simulink model "signalSim"  (R2023b)
settings: Solver=VariableStepAuto  StartTime=0.0  StopTime=0.1  RelTol=1e-3
values from neighbouring files (symbols this model uses):
  f = 1000    [data_gen.m]    (also in test.m = 100)
  fdac = 20e6    (= 20000000)    [data_gen.m]
  fs = 1e6    (= 1000000)    [data_gen.m]    (also in test.m = 1000)
  inc_1e5 = round((100000*2^N)/fdac)    [data_gen.m]
libraries: hdlsllib x3, dspsrcs4 x2, dspfdesign x1, dsphdlsigops2 x1
settings Model: Creator=31651  LastModifiedBy=31651
settings OptimizationCC: BlockReduction=off  ConditionallyExecuteInputs=off

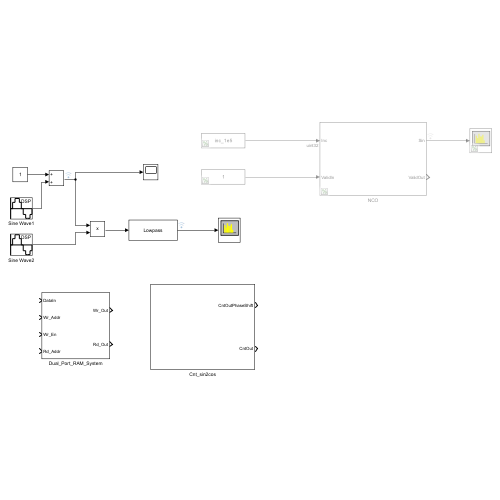
[thumbnail: Simulink's stored preview of the top-level diagram]
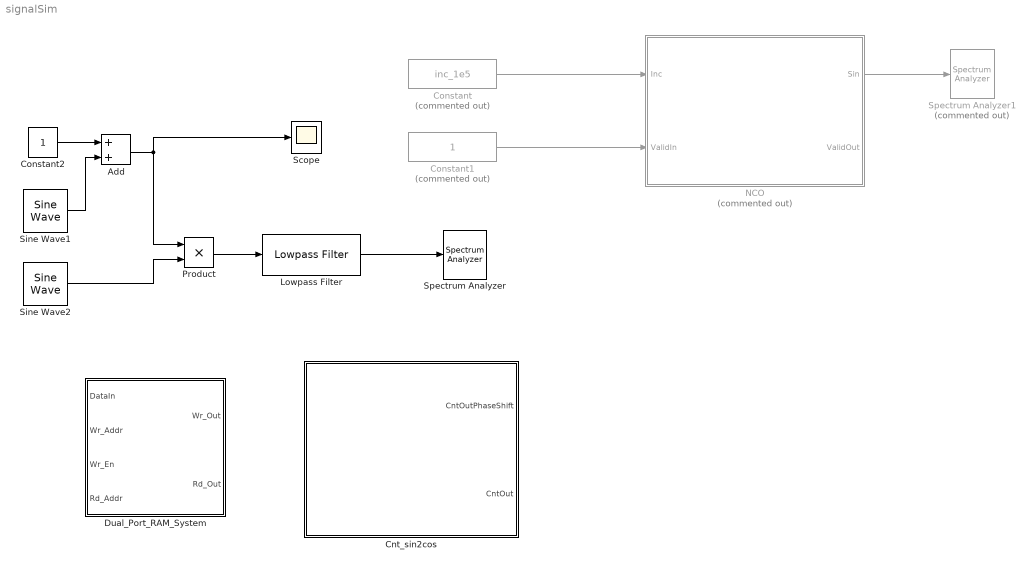
== system signalSim ==
  Add : Sum
  Cnt_sin2cos : Subsystem
  Constant : Constant  Commented=on  Value=inc_1e5  OutDataTypeStr=uint32  SampleTime=1/fdac
  Constant1 : Constant  Commented=on  OutDataTypeStr=boolean  SampleTime=1/fdac
  Constant2 : Constant  SampleTime=1/fs
  Dual_Port_RAM_System : Subsystem
  Lowpass Filter : dspfdesign/Lowpass Filter  FilterType=FIR  DesignForMinimumOrder=on  FilterOrder=50  PassbandFrequency=500  StopbandFrequency=1500  PassbandRipple=0.1  StopbandAttenuation=80  SampleRateMode=Specify on dialog  SampleRate=fs  SimulateUsing=Interpreted execution  roundingMode=Floor  coeffsDataTypeStr=fixdt(1,16)
  NCO : Subsystem  Commented=on
  Product : Product
  Scope : Scope
  Sine Wave1 : dspsrcs4/Sine Wave  Amplitude=1  Frequency=f  Phase=pi/2  SampleMode=Discrete  OutComplex=Real  CompMethod=Trigonometric fcn  TableSize=Speed  SampleTime=1/fs  SamplesPerFrame=1  ResetState=Restart at time zero  OutputFrames=off  dataType=double  wordLen=16  udDataType=sfix(16)  fracBitsMode=Best precision  numFracBits=15  OutDataTypeStr=double  LastOutDataTypeStr=double
  Sine Wave2 : dspsrcs4/Sine Wave  Amplitude=1  Frequency=f  Phase=-pi/6  SampleMode=Discrete  OutComplex=Real  CompMethod=Trigonometric fcn  TableSize=Speed  SampleTime=1/fs  SamplesPerFrame=1  ResetState=Restart at time zero  OutputFrames=off  dataType=double  wordLen=16  udDataType=sfix(16)  fracBitsMode=Best precision  numFracBits=15  OutDataTypeStr=double  LastOutDataTypeStr=double
  Spectrum Analyzer : SpectrumAnalyzer  WindowPosition=[450.000000,323.000000,800.000000,500.000000,]  Visible=on  ScopeFrameLocation=window  Span=1000000  StartFrequency=-500000  StopFrequency=500000  YLimits=[-184.42039117,53.77493033]
  Spectrum Analyzer1 : SpectrumAnalyzer  Commented=on  WindowPosition=[264.000000,231.000000,800.000000,500.000000,]  ScopeFrameLocation=window  YLimits=[-135.03922984,41.64810812]  SelectedToolstripTab=spectrumAnalyzerToolstrip.measurementsTab
  wires:
  Sine Wave2/1 -> Product/2
  Product/1 -> Lowpass Filter/1
  Lowpass Filter/1 -> Spectrum Analyzer/1
  Constant1/1 -> NCO/2(ValidIn)
  NCO/1(Sin) -> Spectrum Analyzer1/1
  Constant/1 -> NCO/1(Inc)
  Constant2/1 -> Add/1
  Sine Wave1/1 -> Add/2
  Add/1 -> Scope/1, Product/1

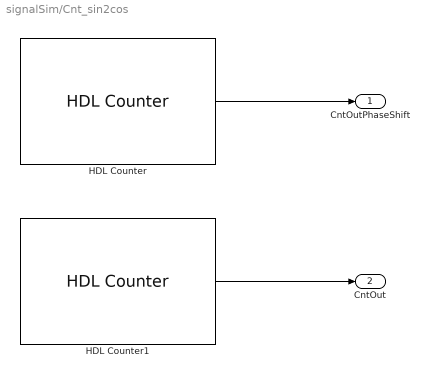
== system signalSim/Cnt_sin2cos ==
  HDL Counter : hdlsllib/Sources/HDL Counter  CountType=Count limited  CountInit=25  CountStep=1  CountMax=1000  CountFromType=Specify  CountFrom=1  CountResetPort=off  CountLoadPort=off  CountEnbPort=off  CountDirPort=off  CountHitOutputPort=off  CountDataType=Unsigned  CountWordLen=16  CountFracLen=0  CountSampTime=1
  HDL Counter1 : hdlsllib/Sources/HDL Counter  CountType=Count limited  CountInit=1  CountStep=1  CountMax=1000  CountFromType=Specify  CountFrom=1  CountResetPort=off  CountLoadPort=off  CountEnbPort=off  CountDirPort=off  CountHitOutputPort=off  CountDataType=Unsigned  CountWordLen=16  CountFracLen=0  CountSampTime=1
  CntOutPhaseShift : Outport  VectorParamsAs1DForOutWhenUnconnected=off
  CntOut : Outport  Port=2  VectorParamsAs1DForOutWhenUnconnected=off
  wires:
  HDL Counter/1 -> CntOutPhaseShift/1
  HDL Counter1/1 -> CntOut/1

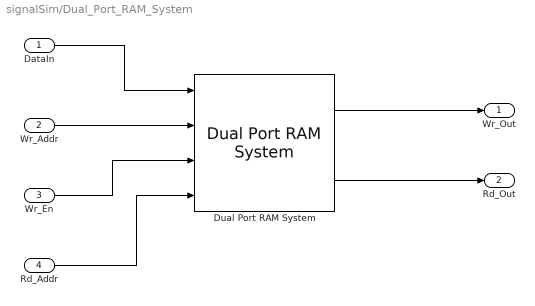
== system signalSim/Dual_Port_RAM_System ==
  DataIn : Inport  OutDataTypeStr=int8
  Wr_Addr : Inport  Port=2  OutDataTypeStr=uint16
  Wr_En : Inport  Port=3  OutDataTypeStr=boolean
  Rd_Addr : Inport  Port=4  OutDataTypeStr=uint16
  Dual Port RAM System : hdlsllib/HDL RAMs/Dual Port RAM System  RAMType=Dual port  AsyncRead=on  WriteOutputValue=New data  RAMInitialValue=0  allowBusInputs=off  WritesHaveOutput=on  NumReads=0  NumWrites=1  SimulateUsing=Code generation
  Wr_Out : Outport  OutDataTypeStr=int8
  Rd_Out : Outport  Port=2  OutDataTypeStr=int8
  wires:
  Wr_En/1 -> Dual Port RAM System/3
  Dual Port RAM System/1 -> Wr_Out/1
  Dual Port RAM System/2 -> Rd_Out/1
  Wr_Addr/1 -> Dual Port RAM System/2
  DataIn/1 -> Dual Port RAM System/1
  Rd_Addr/1 -> Dual Port RAM System/4

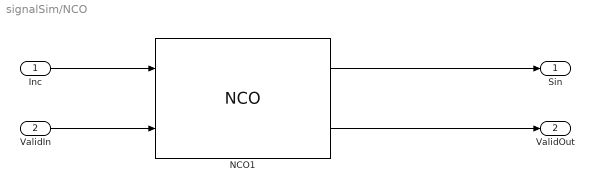
== system signalSim/NCO ==
  Inc : Inport  OutDataTypeStr=uint32
  ValidIn : Inport  Port=2
  NCO1 : dsphdlsigops2/NCO  PhaseIncrementSource=Input port  PhaseIncrement=inc_1e5  PhaseOffsetSource=Property  PhaseOffset=0  DitherSource=Property  NumDitherBits=4  SamplesPerFrame=1  LUTCompress=off  ResetAction=off  Waveform=Sine  PhasePort=off  SimulateUsing=Code generation  AccumulatorWL=N  PhaseQuantization=on  NumQuantizerAccumulatorBits=12  OutputDataType=Binary point scaling  OutputWL=16  OutputFL=14
  Sin : Outport
  ValidOut : Outport  Port=2
  wires:
  NCO1/2 -> ValidOut/1
  NCO1/1 -> Sin/1
  Inc/1 -> NCO1/1
  ValidIn/1 -> NCO1/2
